simulink model "audiointerface1"  (R2021a)
settings: Solver=VariableStepAuto  StartTime=0.0  StopTime=60  RelTol=1e-3
libraries: audiosources x2, dspsnks4 x1, dspsigops x1, dspspect3 x1
settings Model: Creator=vpixx  LastModifiedBy=vpixx

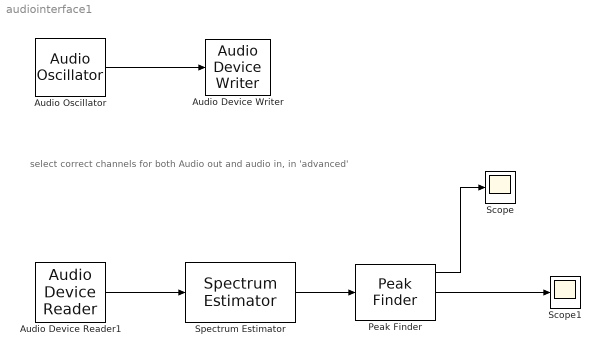
== system audiointerface1 ==
  note: select correct channels for both Audio out and audio in, in 'advanced'
  Audio Device Reader1 : audiosources/Audio Device Reader  Driver=ASIO  Device=Default  SampleRate=192000  NumChannels=8  SamplesPerFrame=1024  BitDepth=16-bit integer  NumBuffers=10  DefaultInputChannelMapping=off  InputChannelMapping=1  OutputNumOverrunSamples=off  OutputDataType=double  DriverIdx=3  DeviceWarnFlag=''
      settings: SourceProductBaseCode=AU
  Audio Device Writer : dspsnks4/Audio Device Writer  Driver=ASIO  Device=M-Audio AIR 192 14 ASIO  InheritSampleRate=off  SampleRate=192000  BitDepth=16-bit integer  BufferSize=4096  NumBuffers=10  DefaultOutputChannelMapping=off  OutputChannelMapping=1  OutputNumUnderrunSamples=off  DriverIdx=3  DeviceWarnFlag=''
  Audio Oscillator : audiosources/Audio Oscillator  FrequencyPort=off  Frequency=18000  AmplitudePort=off  Amplitude=1  DCOffsetPort=off  PhaseOffset=0  DCOffset=0  WidthPort=off  Width=1  DutyCyclePort=off  DutyCycle=0.5  SampsPerFrame=1024  Fs=192000  OutputDataType=double  SimulateUsing=Code generation
      settings: SourceProductBaseCode=AU  SignalType=sine
  Peak Finder : dspsigops/Peak Finder  polarity=Maxima and Minima  indexBase=Zero  outputIdx=off  outputVal=on  maxPeaks=3  NoiseDistinguish=off  thresh=0  roundingMode=Floor  overflowMode=off
      settings: SourceProductBaseCode=DS  allowOverrides=off
  Scope : Scope
  Scope1 : Scope
  Spectrum Estimator : dspspect3/Spectrum Estimator  Method=Welch  NumTapsPerBand=12  SpectrumType=Power  FrequencyResolutionMethod=Auto  FilterBankResolutionMethod=Auto  RBW=5  WindowLength=1024  FrequencyBandsSource=Same as input frame size  FrequencyBands=1024  FFTLengthSource=Auto  FFTLength=1024  InheritSampleRate=on  SampleRate=192000  Window=Hann  SidelobeAttenuation=60  AveragingMethod=Running  SpectralAverages=1  ForgettingFactorPort=off  ForgettingFactor=0.9  Overlap=0  ReferenceLoad=1  FrequencyRange=Centered  PowerUnits=dBm  OutputMaxHoldSpectrum=off  OutputMinHoldSpectrum=off  OutputFrequencyVector=off  OutputRBW=off  SimulateUsing=Code generation
      settings: SourceProductBaseCode=DS
  wires:
  Audio Oscillator/1 -> Audio Device Writer/1
  Audio Device Reader1/1 -> Spectrum Estimator/1
  Spectrum Estimator/1 -> Peak Finder/1
  Peak Finder/1 -> Scope/1
  Peak Finder/2 -> Scope1/1
